simulink model "ActiveSuspensionUsing LQR_simulink"  (R2021a)
settings: Solver=ode1  StartTime=0.0  StopTime=Sim_Time  FixedStep=0.001  RelTol=1e-3
values from neighbouring files (symbols this model uses):
  A = [ 0 1 0 -1 ... (first row only)    [ActiveSuspensionUsing LQR_code.m]
  B = [0  0 ... (first row only)    [ActiveSuspensionUsing LQR_code.m]
  C = [ 1 0 0 0 ... (first row only)    [ActiveSuspensionUsing LQR_code.m]
  D = [0 0 ... (first row only)    [ActiveSuspensionUsing LQR_code.m]
  K = lqr( A, B(:,2), Q, R )    [ActiveSuspensionUsing LQR_code.m]
settings Model: Creator=ku53058  LastModifiedBy=ASUS
settings SolverCC: AlgebraicLoopSolver=TrustRegion
settings DataIOCC: ReturnWorkspaceOutputs=off
settings OptimizationCC: LifeSpan=inf
settings DebuggingCC: SFMachineParentedDataDiag=warning  ArithmeticOperatorsInVariantConditions=warning
settings SFSimCC: SimUseLocalCustomCode=off  CustomCodeUndefinedFunction=UseInterfaceOnly
settings RTWCC: RTWUseLocalCustomCode=off
settings CodeAppCC: StateflowObjectComments=on

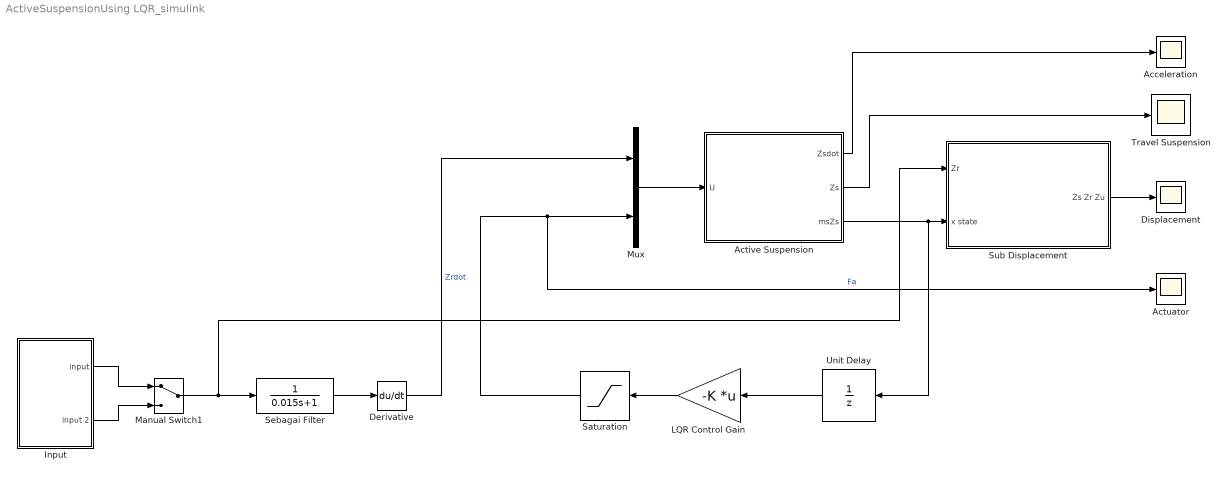
== system ActiveSuspensionUsing LQR_simulink ==
  "Acceleration " : Scope
  Active Suspension : Subsystem
  Actuator : Scope
  Derivative : Derivative
  Displacement : Scope
  Input : Subsystem
  LQR Control Gain : Gain  Gain=-K  Multiplication=Matrix(K*u)
  Manual Switch1 : ManualSwitch
  Mux : Mux  Inputs=2
  Saturation : Saturate  UpperLimit=46730  LowerLimit=-46730
  Sebagai Filter : TransferFcn  Denominator=[0.015 1]
  Sub Displacement : Subsystem
  Travel Suspension : Scope
  Unit Delay : UnitDelay  SampleTime=-1  HasFrameUpgradeWarning=on
  wires:
  LQR Control Gain/1 -> Saturation/1
  Manual Switch1/1 -> Sebagai Filter/1, Sub Displacement/1(Zr)
  Unit Delay/1 -> LQR Control Gain/1
  Saturation/1 -> Mux/2, Actuator/1  "Fa"
  Mux/1 -> Active Suspension/1(U)
  Active Suspension/1(Zsdot) -> "Acceleration "/1
  Active Suspension/2(Zs) -> Travel Suspension/1
  Active Suspension/3(msZs) -> Sub Displacement/2(x state), Unit Delay/1
  Sub Displacement/1(Zs Zr Zu) -> Displacement/1
  Input/1(input) -> Manual Switch1/1
  Input/2(input 2) -> Manual Switch1/2
  Derivative/1 -> Mux/1  "Zrdot"
  Sebagai Filter/1 -> Derivative/1

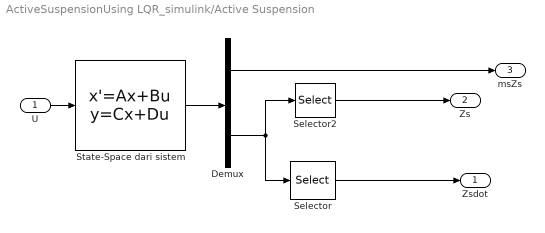
== system ActiveSuspensionUsing LQR_simulink/Active Suspension ==
  U : Inport
  Demux : Demux  Outputs=[4 2]
  Selector : Selector  InputPortWidth=2  IndexOptions=Index vector (dialog)  Indices=[2]  OutputSizes=1
  Selector2 : Selector  InputPortWidth=2  IndexOptions=Index vector (dialog)  Indices=[1]  OutputSizes=1
  State-Space dari sistem : StateSpace  A=A  B=B  C=cat(1,eye(4), C)  D=D  InitialCondition=0
  Zsdot : Outport
  Zs : Outport  Port=2
  msZs : Outport  Port=3
  wires:
  Demux/1 -> msZs/1
  State-Space dari sistem/1 -> Demux/1
  Demux/2 -> Selector2/1, Selector/1
  Selector/1 -> Zsdot/1
  Selector2/1 -> Zs/1
  U/1 -> State-Space dari sistem/1

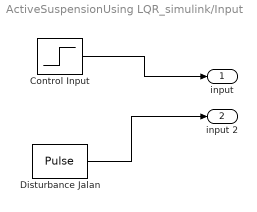
== system ActiveSuspensionUsing LQR_simulink/Input ==
  Control Input : Step  After=0.06  SampleTime=0
  Disturbance Jalan : DiscretePulseGenerator  PulseType=Time based  Amplitude=0.1  Period=6  PulseWidth=50  PhaseDelay=.1
  input : Outport
  input 2 : Outport  Port=2
  wires:
  Disturbance Jalan/1 -> input 2/1
  Control Input/1 -> input/1

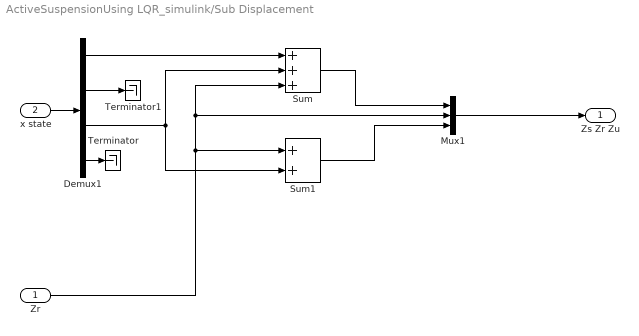
== system ActiveSuspensionUsing LQR_simulink/Sub Displacement ==
  Zr : Inport
  x state : Inport  Port=2
  Demux1 : Demux
  Mux1 : Mux  Inputs=3
  Sum : Sum  Inputs=+++
  Sum1 : Sum
  Terminator : Terminator
  Terminator1 : Terminator
  Zs Zr Zu : Outport
  wires:
  x state/1 -> Demux1/1
  Demux1/2 -> Terminator1/1
  Demux1/4 -> Terminator/1
  Demux1/1 -> Sum/1
  Demux1/3 -> Sum1/2, Sum/2
  Sum/1 -> Mux1/1
  Sum1/1 -> Mux1/3
  Mux1/1 -> Zs Zr Zu/1
  Zr/1 -> Sum1/1, Mux1/2, Sum/3
